simulink model "speedControllerTune"  (R2025b)
settings: Solver=FixedStepAuto  StartTime=0.0  StopTime=10  FixedStep=1e-3  RelTol=1e-3
settings Model: DataDictionary=motorData.sldd  PauseTimes=0.13  Creator=karadeli  LastModifiedBy=karadeli

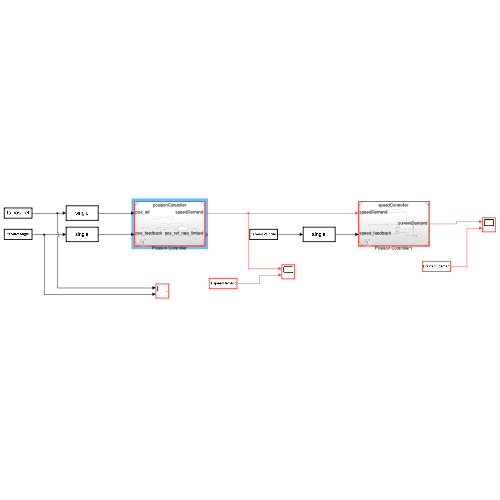
[thumbnail: Simulink's stored preview of the top-level diagram]
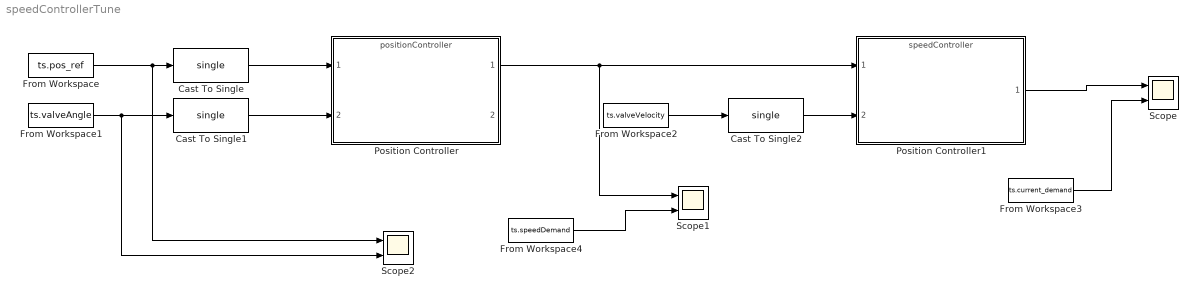
== system speedControllerTune ==
  Cast To Single : DataTypeConversion  OutDataTypeStr=single  SaturateOnIntegerOverflow=off  RndMeth=Floor
  Cast To Single1 : DataTypeConversion  OutDataTypeStr=single  SaturateOnIntegerOverflow=off  RndMeth=Floor
  Cast To Single2 : DataTypeConversion  OutDataTypeStr=single  SaturateOnIntegerOverflow=off  RndMeth=Floor
  From Workspace : FromWorkspace  VariableName=ts.pos_ref
  From Workspace1 : FromWorkspace  VariableName=ts.valveAngle
  From Workspace2 : FromWorkspace  VariableName=ts.valveVelocity
  From Workspace3 : FromWorkspace  VariableName=ts.current_demand  SampleTime=1e-3
  From Workspace4 : FromWorkspace  VariableName=ts.speedDemand  SampleTime=1e-3
  Position Controller : ModelReference  ModelNameDialog=positionController.slx  SimulationMode=Normal  ModelReferenceVersion=1.39
  Position Controller1 : ModelReference  ModelNameDialog=speedController.slx  SimulationMode=Normal  ModelReferenceVersion=1.6
  Scope : Scope  NumInputPorts=2
      settings: ActiveDisplayYMinimum=7.090592794828801  ActiveDisplayYMaximum=14.89629504761856
  Scope1 : Scope  NumInputPorts=2
      settings: ActiveDisplayYMinimum=-3000  ActiveDisplayYMaximum=3000
  Scope2 : Scope  NumInputPorts=2
      settings: ActiveDisplayYMinimum=-1  ActiveDisplayYMaximum=1  DataLoggingVariableName=ScopeData2
  wires:
  Position Controller/1 -> Scope1/1, Position Controller1/1
  From Workspace/1 -> Scope2/1, Cast To Single/1
  From Workspace1/1 -> Scope2/2, Cast To Single1/1
  From Workspace2/1 -> Cast To Single2/1
  Cast To Single/1 -> Position Controller/1
  Cast To Single1/1 -> Position Controller/2
  Cast To Single2/1 -> Position Controller1/2
  Position Controller1/1 -> Scope/1
  From Workspace3/1 -> Scope/2
  From Workspace4/1 -> Scope1/2
